simulink model "tf_block"  (R2016a)
settings: Solver=FixedStepDiscrete  StartTime=0.0  StopTime=10.0  RelTol=1e-3
undefined symbols (not defined in the file): a1, a2, a3, a4, a5, a6
libraries: simulink x1
settings Model: Creator=Admin  LastModifiedBy=Admin

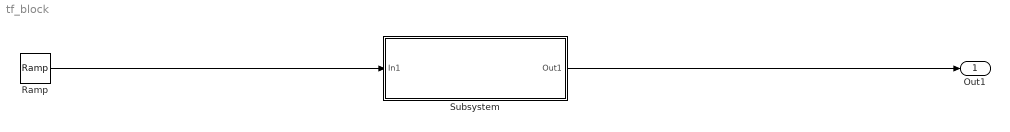
== system tf_block ==
  Ramp : simulink/Sources/Ramp  slope=1  start=0  X0=0
  Subsystem : Subsystem
  Out1 : Outport
  wires:
  Ramp/1 -> Subsystem/1(In1)
  Subsystem/1(Out1) -> Out1/1

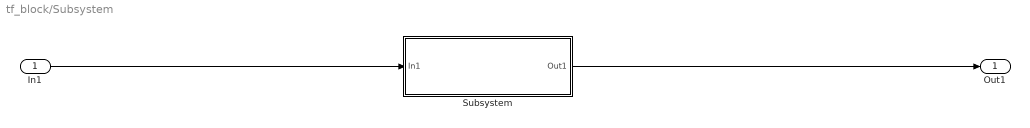
== system tf_block/Subsystem ==
  In1 : Inport
  Subsystem : Subsystem
  Out1 : Outport
  wires:
  In1/1 -> Subsystem/1(In1)
  Subsystem/1(Out1) -> Out1/1

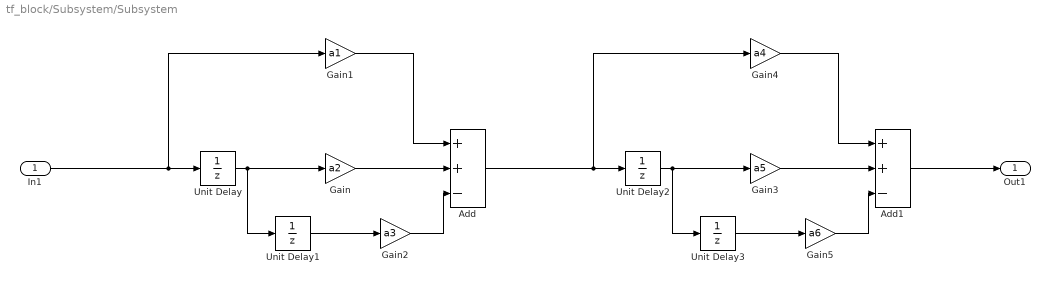
== system tf_block/Subsystem/Subsystem ==
  In1 : Inport
  Add : Sum  Inputs=++-
  Add1 : Sum  Inputs=++-
  Gain : Gain  Gain=a2
  Gain1 : Gain  Gain=a1
  Gain2 : Gain  Gain=a3
  Gain3 : Gain  Gain=a5
  Gain4 : Gain  Gain=a4
  Gain5 : Gain  Gain=a6
  Unit Delay{,1..3} (4 alike) : UnitDelay  SampleTime=-1
  Out1 : Outport
  wires:
  Unit Delay/1 -> Unit Delay1/1, Gain/1
  Gain1/1 -> Add/1
  In1/1 -> Unit Delay/1, Gain1/1
  Add1/1 -> Out1/1
  Gain3/1 -> Add1/2
  Gain2/1 -> Add/3
  Unit Delay1/1 -> Gain2/1
  Add/1 -> Unit Delay2/1, Gain4/1
  Unit Delay3/1 -> Gain5/1
  Unit Delay2/1 -> Unit Delay3/1, Gain3/1
  Gain/1 -> Add/2
  Gain5/1 -> Add1/3
  Gain4/1 -> Add1/1
